simulink model "Ball"  (Simulink 9.1)
settings: Solver=ode45  StartTime=0.0  StopTime=20  MaxStep=0.01  RelTol=1e-3
settings Model: Creator=Asus  LastModifiedBy=Asus
settings DataIOCC: SaveFormat=Dataset
settings OptimizationCC: LifeSpan=auto
settings DebuggingCC: UnderspecifiedInitializationDetection=Simplified  MergeDetectMultiDrivingBlocksExec=error  SFUnexpectedBacktrackingDiag=error  SFNoUnconditionalDefaultTransitionDiag=error  SFExecutionAtInitializationDiag=warning
settings HardwareCC: ProdBitPerPointer=64  ProdBitPerSizeT=64  ProdBitPerPtrDiffT=64  ProdLargestAtomicFloat=Float  ProdIntDivRoundTo=Zero  ProdEndianess=LittleEndian  ProdWordSize=64  ProdHWDeviceType=Intel->x86-64 (Windows64)
settings ModelReferenceCC: PropagateSignalLabelsOutOfModel=on
settings CodeAppCC: StateflowObjectComments=off
settings GRTTargetCC: TargetLangStandard=C99 (ISO)  CombineOutputUpdateFcns=on  GRTInterface=off
settings ConfigComp: CovMetricSettings=dwe  CovHtmlReporting=off  CovSaveCumulativeToWorkspaceVar=off  CovSaveSingleToWorkspaceVar=off  CovExternalEMLEnable=on

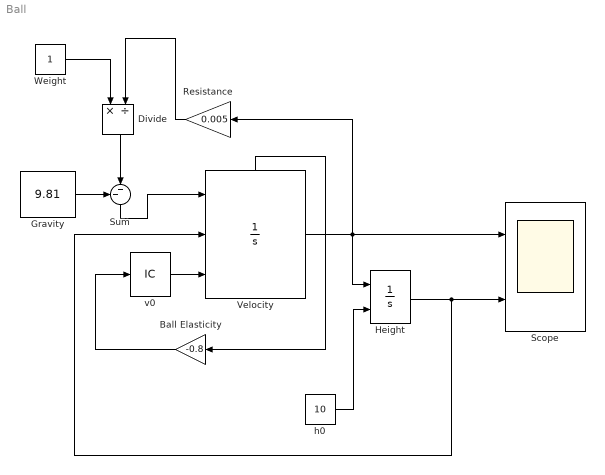
== system Ball ==
  Ball Elasticity : Gain  Gain=-0.8
  Divide : Product  Inputs=*/
  "Gravity " : Constant  Value=9.81
  "Height " : Integrator  InitialConditionSource=external  LimitOutput=on  LowerSaturationLimit=0
  Resistance : Gain  Gain=0.005
  Scope : Scope  NumInputPorts=2
  Sum : Sum  Inputs=--|
  Velocity : Integrator  ExternalReset=falling  InitialConditionSource=external  ShowStatePort=on
  Weight : Constant
  "h0 " : Constant  Value=10
  v0 : InitialCondition  Value=15
  wires:
  "Gravity "/1 -> Sum/1
  Sum/1 -> Velocity/1
  "Height "/1 -> Velocity/2, Scope/2
  Velocity/1 -> Resistance/1, "Height "/1, Scope/1
  "h0 "/1 -> "Height "/2
  v0/1 -> Velocity/3
  Ball Elasticity/1 -> v0/1
  Velocity/State -> Ball Elasticity/1
  Resistance/1 -> Divide/2
  Weight/1 -> Divide/1
  Divide/1 -> Sum/2
